simulink model "ControlMultiV1_1"  (R2015b)
settings: Solver=ode1  StartTime=0.0  StopTime=inf  FixedStep=0.001  RelTol=1e-3
libraries: simulink x2
settings Model: ExtModeTrigDuration=10000  Creator=ale  LastModifiedBy=anle
settings SolverCC: PositivePriorityOrder=on
settings RTWCC: SystemTargetFile=quarc_linux_duovero.tlc  TemplateMakefile=quarc_linux_duovero_tmf  Description=QUARC Linux DuoVero Target (QBall 2, QBot 2)
settings STFCustomTargetCC: TargetLibSuffix=.a  TargetPreCompLibLocation=C:\PROGRA~3\QUARC\lib\2015b\LINUX_~1\release  GeneratePreprocessorConditionals=Use local settings  CPPClassGenCompliant=off  SystemTargetFile=quarc_linux_duovero.tlc
settings GRTTargetCC: TargetLibSuffix=.a  TargetPreCompLibLocation=C:\PROGRA~3\QUARC\lib\2015b\LINUX_~1\release  ParMdlRefBuildCompliant=off  CompOptLevelCompliant=off  CombineOutputUpdateFcns=off  MatFileLogging=off  CPPClassGenCompliant=off  GRTInterface=on  UseToolchainInfoCompliant=off  ExtMode=on  ExtModeMexFile=quarc_comm  ExtModeMexArgs='-w -d /tmp -uri %u'

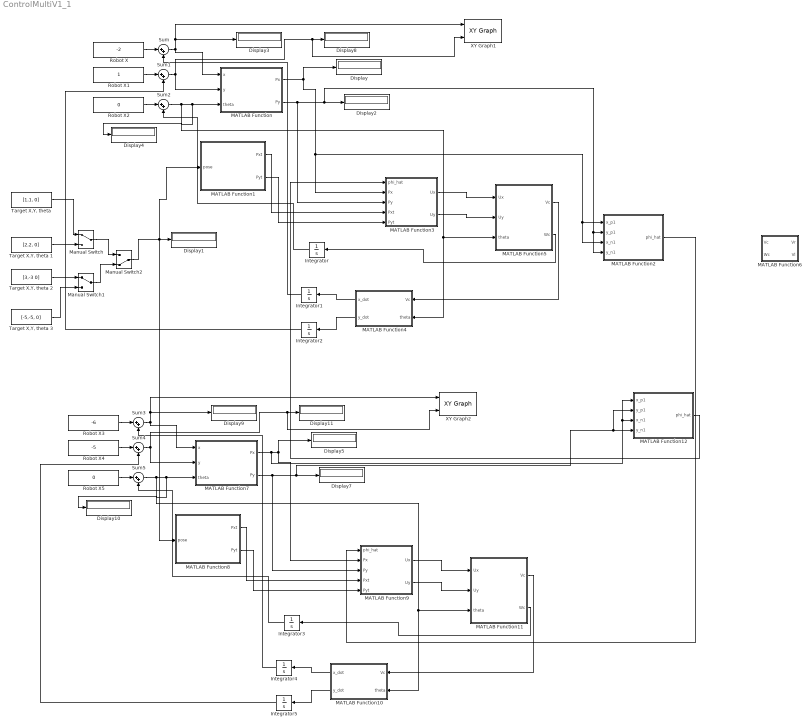
== system ControlMultiV1_1 ==
  Display{,1..5,7..11} (11 alike) : Display
  Integrator{,1..5} (6 alike) : Integrator
  MATLAB Function : MATLAB Function  TreatAsAtomicUnit=on
  MATLAB Function1 : MATLAB Function  TreatAsAtomicUnit=on
  MATLAB Function10 : MATLAB Function  TreatAsAtomicUnit=on
  MATLAB Function11 : MATLAB Function  TreatAsAtomicUnit=on
  MATLAB Function12 : MATLAB Function  TreatAsAtomicUnit=on
  MATLAB Function2 : MATLAB Function  TreatAsAtomicUnit=on
  MATLAB Function3 : MATLAB Function  TreatAsAtomicUnit=on
  MATLAB Function4 : MATLAB Function  TreatAsAtomicUnit=on
  MATLAB Function5 : MATLAB Function  TreatAsAtomicUnit=on
  MATLAB Function6 : MATLAB Function  TreatAsAtomicUnit=on
  MATLAB Function7 : MATLAB Function  TreatAsAtomicUnit=on
  MATLAB Function8 : MATLAB Function  TreatAsAtomicUnit=on
  MATLAB Function9 : MATLAB Function  TreatAsAtomicUnit=on
  Manual Switch : ManualSwitch
  Manual Switch1 : ManualSwitch
  Manual Switch2 : ManualSwitch  CurrentSetting=0
  Robot X : Constant  Value=-2
  Robot X1 : Constant
  Robot X2 : Constant  Value=0
  Robot X3 : Constant  Value=-6
  Robot X4 : Constant  Value=-5
  Robot X5 : Constant  Value=0
  Sum{,1..5} (6 alike) : Sum  Inputs=|++
  "Target X,Y, theta " : Constant  Value=[1,1, 0]
  "Target X,Y, theta 1" : Constant  Value=[2,2, 0]
  "Target X,Y, theta 2" : Constant  Value=[3,-3 0]
  "Target X,Y, theta 3" : Constant  Value=[-5,-5, 0]
  XY Graph1 : simulink/Sinks/XY Graph  xmin=-20  xmax=20  ymin=-20  ymax=20  st=-1
  XY Graph2 : simulink/Sinks/XY Graph  xmin=-20  xmax=20  ymin=-20  ymax=20  st=-1
  wires:
  MATLAB Function1/1(Pxt) -> MATLAB Function3/4(Pxt)
  MATLAB Function1/2(Pyt) -> MATLAB Function3/5(Pyt)
  MATLAB Function/2(Py) -> MATLAB Function3/3(Py), MATLAB Function2/4(y_n1), MATLAB Function2/2(y_p1), Display2/1
  MATLAB Function/1(Px) -> MATLAB Function2/3(x_n1), MATLAB Function2/1(x_p1), MATLAB Function3/2(Px), Display/1
  Sum2/1 -> MATLAB Function4/2(theta), MATLAB Function5/3(theta), Display4/1, MATLAB Function/3(theta)
  Sum1/1 -> MATLAB Function/2(y), XY Graph1/2, Display8/1
  Sum/1 -> MATLAB Function/1(x), XY Graph1/1, Display3/1
  Robot X2/1 -> Sum2/1
  Robot X/1 -> Sum/1
  Robot X1/1 -> Sum1/1
  Manual Switch2/1 -> MATLAB Function8/1(pose), MATLAB Function1/1(pose), Display1/1
  "Target X,Y, theta "/1 -> Manual Switch/1
  "Target X,Y, theta 1"/1 -> Manual Switch/2
  Manual Switch/1 -> Manual Switch2/1
  Manual Switch1/1 -> Manual Switch2/2
  "Target X,Y, theta 2"/1 -> Manual Switch1/1
  "Target X,Y, theta 3"/1 -> Manual Switch1/2
  MATLAB Function3/1(Ux) -> MATLAB Function5/1(Ux)
  MATLAB Function3/2(Uy) -> MATLAB Function5/2(Uy)
  MATLAB Function5/1(Vc) -> MATLAB Function4/1(Vc)
  MATLAB Function5/2(Wc) -> Integrator/1
  Integrator/1 -> Sum2/2
  MATLAB Function4/1(x_dot) -> Integrator1/1
  Integrator1/1 -> Sum/2
  MATLAB Function4/2(y_dot) -> Integrator2/1
  Integrator2/1 -> Sum1/2
  MATLAB Function8/1(Pxt) -> MATLAB Function9/4(Pxt)
  MATLAB Function8/2(Pyt) -> MATLAB Function9/5(Pyt)
  MATLAB Function7/2(Py) -> MATLAB Function9/3(Py), MATLAB Function12/2(y_p1), MATLAB Function12/4(y_n1), Display7/1
  MATLAB Function7/1(Px) -> MATLAB Function12/3(x_n1), MATLAB Function12/1(x_p1), MATLAB Function9/2(Px), Display5/1
  Sum5/1 -> MATLAB Function10/2(theta), MATLAB Function11/3(theta), Display10/1, MATLAB Function7/3(theta)
  Sum4/1 -> MATLAB Function7/2(y), XY Graph2/2, Display11/1
  Sum3/1 -> MATLAB Function7/1(x), XY Graph2/1, Display9/1
  Robot X5/1 -> Sum5/1
  Robot X3/1 -> Sum3/1
  Robot X4/1 -> Sum4/1
  MATLAB Function9/1(Ux) -> MATLAB Function11/1(Ux)
  MATLAB Function9/2(Uy) -> MATLAB Function11/2(Uy)
  MATLAB Function11/1(Vc) -> MATLAB Function10/1(Vc)
  MATLAB Function11/2(Wc) -> Integrator3/1
  Integrator3/1 -> Sum5/2
  MATLAB Function10/1(x_dot) -> Integrator4/1
  Integrator4/1 -> Sum3/2
  MATLAB Function10/2(y_dot) -> Integrator5/1
  Integrator5/1 -> Sum4/2
  MATLAB Function12/1(phi_hat) -> MATLAB Function3/1(phi_hat)
  MATLAB Function2/1(phi_hat) -> MATLAB Function9/1(phi_hat)

== matlab function ControlMultiV1_1/MATLAB Function1 ==
  data: pose input; Pxt output; Pyt output
function [Pxt,Pyt] = PxtPyt_convert(pose)
x=pose(1);
y=pose(2);
theta=pose(2);
l=.0235; %#length between the two wheels in meters
%R=.0175; %#R or signed distance from ICC (Instanteous center of curvature) in meters
Pxt= x+l*cos(theta)
Pyt = y+l*sin(theta)

%#codegen

== matlab function ControlMultiV1_1/MATLAB Function ==
  data: x input; Px output; Py output; y input; theta input
function [Px,Py] = PxPy_convert(x, y, theta)

l=.0235; %#length between the two wheels in meters
%R=.0175; %#R or signed distance from ICC (Instanteous center of curvature) in meters
Px= x+l*cos(theta)
Py = y+l*sin(theta)

%#codegen

== matlab function ControlMultiV1_1/MATLAB Function2 ==
  data: x_p1 input; phi_hat output; y_p1 input; x_n1 input; y_n1 input
function phi_hat  = rho_phi_convert(x_p1,y_p1,x_n1,y_n1)
%x_p1,y_p1,x_n1,y_n1 are for phi_i+1, phi_i-1

[phi_p1, rho] = cart2pol((x_p1),(y_p1))

[phi_n1, rho] = cart2pol((x_n1),(y_n1))

phi_hat = (phi_p1+phi_n1+2*pi)/2

== matlab function ControlMultiV1_1/MATLAB Function3 ==
  data: phi_hat input; Px input; Ux output; Py input; Pxt input; Pyt input; Uy output
function [Ux, Uy] = UxUy(phi_hat,Px,Py,Pxt,Pyt)
%#codegen
%rho_star=.5;
%omega_star=.5;
 
krho = 0.5;
kphi = 1;
w_d=1;
 
U = [0 0];
rho_size = 1;
phi_size = 1;
[phi, rho] = cart2pol(Px,Py);
[phi_d, rho_d] = cart2pol(Pxt,Pyt);
 
[phi_dif, rho_dif] = cart2pol((Px-Pxt),(Py-Pyt));
 
PxD = Px - Pxt; 
PyD = Py - Pyt;
 
 
 
J_i=[PxD/(sqrt(PxD^2+PyD^2)) PyD/(sqrt(PxD^2+PyD^2)); -PyD/(PxD^2+PyD^2) PxD/(PxD^2+PyD^2)];
 
 
 
 
%J_i=[(Px-Pxt)/phi_dif (Py-Pyt)/phi_dif;...
%    -(Py-Pyt)/((1+((Py-Pyt)/(PD))^2)*(Px-Pxt)^2)  1/((1+((Py-Pyt)/(PD))^2)*(Px-Pxt))];
 
 
 
%J_i=[ (Px-Pxt)/phi (Py-Pyt)/phi_dif;    -(Py-Pyt)/(phi_dif)^2  (Px-Pxt)/(phi_dif)^2 ];
 
rhoi_dot = krho*(rho_size-rho_dif)
phii_dot = w_d + kphi*(phi_hat-phi);
V_i= [rhoi_dot; phii_dot];
Rt = [ 1 0; 0 1];
 
 
U = Rt*(J_i'*V_i);
U = inv(J_i)*V_i; 
Ux = U(1);
Uy = U(2);

== matlab function ControlMultiV1_1/MATLAB Function4 ==
  data: Vc input; x_dot output; theta input; y_dot output
function [x_dot, y_dot] = VcWc2XYdot(Vc, theta)
%#codegen
x_dot = Vc*cos(theta)
y_dot = Vc*sin(theta)

== matlab function ControlMultiV1_1/MATLAB Function5 ==
  data: Ux input; Vc output; Uy input; Wc output; theta input
function [Vc,Wc] = UxUy2VcWc(Ux,Uy, theta)

l=.0235; %#length between the two wheels in meters
kin_inv = inv([cos(theta) -l*sin(theta) ; sin(theta) l*cos(theta)]);
P =  kin_inv*[Ux;Uy];
Vc=P(1);
Wc=P(2);

== matlab function ControlMultiV1_1/MATLAB Function6 ==
  data: Vc input; Vr output; Wc input; Vl output
function [Vr,Vl] = VcWc2VrVl(Vc,Wc)
%#codegen

l=.0235;
Vr = Vc+(1/2)*(l*2)*Wc;
Vl = Vc-(1/2)*(l*2)*Wc;

== matlab function ControlMultiV1_1/MATLAB Function10 ==
  data: Vc input; x_dot output; theta input; y_dot output
function [x_dot, y_dot] = VcWc2XYdot(Vc, theta)
%#codegen
x_dot = Vc*cos(theta)
y_dot = Vc*sin(theta)

== matlab function ControlMultiV1_1/MATLAB Function11 ==
  data: Ux input; Vc output; Uy input; Wc output; theta input
function [Vc,Wc] = UxUy2VcWc(Ux,Uy, theta)

l=.0235; %#length between the two wheels in meters
kin_inv = inv([cos(theta) -l*sin(theta) ; sin(theta) l*cos(theta)]);
P =  kin_inv*[Ux;Uy];
Vc=P(1);
Wc=P(2);

== matlab function ControlMultiV1_1/MATLAB Function7 ==
  data: x input; Px output; Py output; y input; theta input
function [Px,Py] = PxPy_convert(x, y, theta)

l=.0235; %#length between the two wheels in meters
%R=.0175; %#R or signed distance from ICC (Instanteous center of curvature) in meters
Px= x+l*cos(theta)
Py = y+l*sin(theta)

%#codegen

== matlab function ControlMultiV1_1/MATLAB Function8 ==
  data: pose input; Pxt output; Pyt output
function [Pxt,Pyt] = PxtPyt_convert(pose)
x=pose(1);
y=pose(2);
theta=pose(2);
l=.0235; %#length between the two wheels in meters
%R=.0175; %#R or signed distance from ICC (Instanteous center of curvature) in meters
Pxt= x+l*cos(theta)
Pyt = y+l*sin(theta)

%#codegen

== matlab function ControlMultiV1_1/MATLAB Function9 ==
  data: phi_hat input; Px input; Ux output; Py input; Pxt input; Pyt input; Uy output
function [Ux, Uy] = UxUy(phi_hat,Px,Py,Pxt,Pyt)
%#codegen
%rho_star=.5;
%omega_star=.5;
 
krho = 0.5;
kphi = 1;
w_d=1;
 
U = [0 0];
rho_size = 1;
phi_size = 1;
[phi, rho] = cart2pol(Px,Py);
[phi_d, rho_d] = cart2pol(Pxt,Pyt);
 
[phi_dif, rho_dif] = cart2pol((Px-Pxt),(Py-Pyt));
 
PxD = Px - Pxt; 
PyD = Py - Pyt;
 
 
 
J_i=[PxD/(sqrt(PxD^2+PyD^2)) PyD/(sqrt(PxD^2+PyD^2)); -PyD/(PxD^2+PyD^2) PxD/(PxD^2+PyD^2)];
 
 
 
 
%J_i=[(Px-Pxt)/phi_dif (Py-Pyt)/phi_dif;...
%    -(Py-Pyt)/((1+((Py-Pyt)/(PD))^2)*(Px-Pxt)^2)  1/((1+((Py-Pyt)/(PD))^2)*(Px-Pxt))];
 
 
 
%J_i=[ (Px-Pxt)/phi (Py-Pyt)/phi_dif;    -(Py-Pyt)/(phi_dif)^2  (Px-Pxt)/(phi_dif)^2 ];
 
rhoi_dot = krho*(rho_size-rho_dif)
phii_dot = w_d+ kphi*((phi_hat-phi));
V_i= [rhoi_dot; phii_dot];
Rt = [ 1 0; 0 1];
 
 
U = Rt*(J_i'*V_i);
U = inv(J_i)*V_i; 
Ux = U(1);
Uy = U(2);

== matlab function ControlMultiV1_1/MATLAB Function12 ==
  data: x_p1 input; phi_hat output; y_p1 input; x_n1 input; y_n1 input
function phi_hat  = rho_phi_convert(x_p1,y_p1,x_n1,y_n1)
%x_p1,y_p1,x_n1,y_n1 are for phi_i+1, phi_i-1

[phi_p1, rho] = cart2pol((x_p1),(y_p1))

[phi_n1, rho] = cart2pol((x_n1),(y_n1))

phi_hat = (phi_p1+phi_n1+2*pi)/2
